simulink model "Model"  (R2018b)
settings: Solver=ode1  StartTime=0.0  StopTime=inf  FixedStep=0.5  RelTol=1e-3
PostLoadFcn:
  | if any(exist('dsrtsu_mdlpostloadfcn', 'file') ~= 0), dsrtsu_mdlpostloadfcn('Execute', bdroot); end
InitFcn:
  | , if any(exist('dsmpb_private', 'file') ~= 0), dsmpb_private('dsmpb_mdlclblib', 'Init', bdroot); end,
  | load('LUT_PSM.mat')
  | load('Torque_ts.mat')
  | 
  | p = 1;
  | L_q = 1.575e-3;
  | L_d = L_q;
  | Psi_M = 0.0353*2*pi;
  | R_s = 639e-3;
  | Ts = 1/25e3;
  | J_ges = 9.56e-5;
  | d_viskos = 0.01;
  | mpsTestMaxVelocityDmd = 166.7;
  | mpsTestVelocityDmd = 0;
  | EDC_CURRENT_CONTROL_EXECUTION_PERIOD = 4e-5;
  | 
undefined symbols (not defined in the file): d, motor_KF, Psidq, Psiqd, q
libraries: dsmpblib x12, simulink x1, simulink_extras x1
(part 2 of 2)

== matlab function Model/DIME Regler/Controller/Decoupling ==
  data: iq input; yd output; p input; w input; Lq input; id input; Ld input; yq output; phi input
function [yd,yq] = fcn(iq,p,w,Lq,id,Ld,phi)

yd= -iq*w*p*Lq;

yq= id*w*p*Ld +phi*p*w;

== matlab function Model/DIME Regler/Controller/MATLAB Function ==
  data: T input; iq output
function iq = fcn(T)
p=1;
Psi_M = 0.0353*2*pi;
iq = T/(3/2* p *Psi_M);

== matlab function Model/DIME Regler/Controller/Identifier_AnyTask/NN Identifier ==
  settings: updateMethod=DISCRETE
  data: h input; id input; iq input; ud input; uq input; omega input; R output; d_id input; d_iq input; Gamma_Theta_R input; Gamma_W_R input; psi_m0 output; J output; Gamma_Theta_psi input; Gamma_W_psi input; takeover input; psim0_est input
function [R, psi_m0, J] = Approximate(h,id,iq,ud,uq,omega, d_id, d_iq, ...
    Gamma_Theta_R, Gamma_W_R,  Gamma_Theta_psi, Gamma_W_psi, takeover, psim0_est )

    % % HRB nominal parameters 
    % Psi_M = 0.0353*2*pi;
    % R_s = 639e-3;


 
if(1)
    Gamma_Theta_ldq10=0;
    Gamma_W_ldq10 = 0;
end
if(1)
    Gamma_Theta_lqd10=0;
    Gamma_W_lqd10 = 0;
end
 




persistent W_R_T ...
           W_l_qd10_T ...
           W_l_dq10_T ...
           W_psi_m0_T ...
           Theta_R_T ...
           Theta_l_qd10_T ...
           Theta_l_dq10_T ...
           Theta_psi_m0_T ...


if isempty(W_R_T) || isempty(W_l_qd10_T) || isempty(W_l_dq10_T) ||  isempty(W_psi_m0_T) || isempty(Theta_R_T) || isempty(Theta_l_qd10_T)  || isempty(Theta_l_dq10_T) ||  isempty(Theta_psi_m0_T)      
 
 
W_R_T = [2.04822644461840e-05,2.04816119048058e-05;2.04823577258696e-05,2.04822462184732e-05;2.04815774888327e-05,2.04817617170584e-05;2.04823629611794e-05,2.04819781184588e-05;2.04820849325778e-05,2.04816182220611e-05;2.04815497917300e-05,2.04820542332664e-05;2.04817290895107e-05,2.04817135625764e-05;2.04819978477042e-05,2.04821050452835e-05;2.04824082972273e-05,2.04821400048950e-05;2.04824137487725e-05,2.04821970118301e-05];
 
Theta_R_T = [0.0179437411497698	0.00897193402779521	0.00897193446402229	0.00897193417960009	0.00897193400199923	0.00897193458740008	0.00897193452389927	0.00897193419739507	0.00897193427267327	0.00897193423924112	0.00897193386022727];
 
W_psi_m0_T = [3.36596323929511e-07,3.35943782551311e-07;3.36687643195459e-07,3.36576135799067e-07;3.35908676332707e-07,3.36092904558458e-07;3.36694960020311e-07,3.36310117299679e-07;3.36414284189910e-07,3.35947573673185e-07;3.35879428791493e-07,3.36383870327895e-07;3.36060197795233e-07,3.36044670860906e-07;3.36328623112877e-07,3.36435820692149e-07;3.36739227973001e-07,3.36470935640707e-07;3.36746389889419e-07,3.36529652947043e-07];
 
Theta_psi_m0_T  = [0.00231788201112145	0.00115894119229074	0.00115894162568093	0.00115894134619483	0.00115894116467780	0.00115894175257942	0.00115894168946356	0.00115894136358532	0.00115894143628631	0.00115894140111420	0.00115894102185007];
 
Theta_l_dq10_T = [3.06272108646170e-05	1.53136618898215e-05	1.53140948664430e-05	1.53138161019030e-05	1.53136340111074e-05	1.53142222806330e-05	1.53141592211266e-05	1.53138334334557e-05	1.53139057572415e-05	1.53138703302795e-05	1.53134910283740e-05];
 
Theta_l_qd10_T = [3.61010730022179e-05	2.24659001336882e-05	2.24663328343095e-05	2.24660542446031e-05	2.24658722745621e-05	2.24664601632891e-05	2.24663971440134e-05	2.24660715653744e-05	2.24661438450041e-05	2.24661084424157e-05	2.24657293848019e-05];
 
W_l_dq10_T = [8.14669546231156e-10,1.62128168031204e-10;9.05741112018515e-10,7.94233715626875e-10;1.26933856909712e-10,3.11162082660982e-10;9.13321502492780e-10,5.28478781859986e-10;6.32309396785878e-10,1.65598880060266e-10;9.74900727413724e-11,6.01931609143709e-10;2.78445392179253e-10,2.62918457852358e-10;5.46829246235578e-10,6.54026825507379e-10;9.57454291187415e-10,6.89161958893324e-10;9.64833086769558e-10,7.48096144394093e-10];
 
W_l_qd10_T = [-0.000643412476326285,-0.000643413128867663;-0.000643412385485832,-0.000643412496993229;-0.000643413163888063,-0.000643412979659837;-0.000643412377824077,-0.000643412762666797;-0.000643412658626792,-0.000643413125337309;-0.000643413193414641,-0.000643412688973105;-0.000643413012409694,-0.000643413027936628;-0.000643412744237816,-0.000643412637040237;-0.000643412333756349,-0.000643412602048681;-0.000643412326400265,-0.000643412543137207];


end

 
x=1;    
 

x_bar = [1,x]';


 
L_q = 1.575e-3;
L_d = L_q;



R      = Theta_R_T      * Phi_1_T( W_R_T * x_bar )  ;

l_qd10 = L_q ;

l_dq10 = L_d ;

psi_m0 = Theta_psi_m0_T * Phi_1_T( W_psi_m0_T * x_bar ) ;

if(takeover)
psi_m0=psim0_est;
end

l_dq20 = 0; 
l_dq30 = 0; 
l_qd30 = 0; 
c_dq01 = 0;  
c_dq11 = 0;  

 
 
ud_hat = R*id - omega * ( l_qd10*iq + l_qd30*iq^3 + c_dq01*id*iq + 0.5*c_dq11*id^2*iq ) + (l_dq10 + 2*l_dq20*id + 3*l_dq30*id^2 + 0.5*c_dq11*iq^2) *  d_id;

uq_hat = R*iq + omega * ( psi_m0 + 0.5*c_dq01*iq^2 + l_dq10*id + l_dq20*id^2 + l_dq30*id^3 + 0.5*c_dq11*id*iq^2 ) + ( l_qd10 + 3*l_qd30*iq^2 + c_dq01*id + 0.5*c_dq11*id^2 ) * d_iq;

J = 0.5 * (ud_hat - ud)^2 + 0.5 * (uq_hat - uq)^2 ;

DJd = ud_hat - ud;
DJq = uq_hat - uq;

 


J_Theta_R_T      = Phi_1_T( W_R_T      * x_bar ) * (DJd * id                                   + DJq * iq);
J_Theta_l_qd10_T = Phi_1_T( W_l_qd10_T * x_bar ) * (DJd * (-omega*iq)                          + DJq * d_iq);
J_Theta_l_dq10_T = Phi_1_T( W_l_dq10_T * x_bar ) * (DJd * ( d_id )                             + DJq * ( id )* omega ) ;
J_Theta_psi_m0_T = Phi_1_T( W_psi_m0_T * x_bar ) * (                                             DJq * ( omega ));

  
J_W_R_T      = x_bar *( Theta_R_T(2:end)      * diag( dsigma( W_R_T      * x_bar ) ) * ( DJd * ( id )                                 + DJq * ( iq ) ) ); % 8x1 * 1x3 = 8x3
J_W_l_qd10_T = x_bar *( Theta_l_qd10_T(2:end) * diag( dsigma( W_l_qd10_T * x_bar ) ) * ( DJd * ( -omega*iq )                          + DJq * ( d_iq ) ) ); 
J_W_l_dq10_T = x_bar *( Theta_l_dq10_T(2:end) * diag( dsigma( W_l_dq10_T * x_bar ) ) * ( DJd * ( d_id )                               + DJq * ( omega*id ) ) ); 
J_W_psi_m0_T = x_bar *( Theta_psi_m0_T(2:end) * diag( dsigma( W_psi_m0_T * x_bar ) ) * (                                                DJq * ( omega ) ) ); 


Theta_R_T      = Theta_R_T      - 5e2*Gamma_Theta_R * J_Theta_R_T'      * h; 
Theta_l_qd10_T = Theta_l_qd10_T -  .2*Gamma_Theta_lqd10 * J_Theta_l_qd10_T'    * h; 
Theta_l_dq10_T = Theta_l_dq10_T -  .00005*Gamma_Theta_ldq10 * J_Theta_l_dq10_T' * h; 
Theta_psi_m0_T = Theta_psi_m0_T - 1*Gamma_Theta_psi * J_Theta_psi_m0_T'   * h;  

 
W_R_T      = W_R_T      - 5e2*Gamma_W_lqd10 * J_W_R_T'      * h; 
W_l_qd10_T = W_l_qd10_T - .2*Gamma_W_R * J_W_l_qd10_T' * h; 
W_l_dq10_T = W_l_dq10_T - .00005*Gamma_W_ldq10 * J_W_l_dq10_T' * h; 
W_psi_m0_T = W_psi_m0_T - 1*Gamma_W_psi * J_W_psi_m0_T' * h; 

  
 


 

function ds = dsigma(x)
a = 1;
ds = a*exp(-a*x)./( 1 + exp(-a*x) ).^2;
end

function Sigma = Phi_1_T(x)
a = 1;
s = 1./( 1 + exp(-a*x) );
Sigma = [1;s];
end

 

 


end

== matlab function Model/DIME Regler/Controller/MATLAB Function1 ==
  data: Udc input; Udc_filt output; Udc_set input
function Udc_filt = fcn(Udc, Udc_set)

if abs(Udc - Udc_set) > 20; 
    Udc_filt = Udc_set; 
else Udc_filt = Udc;
end

== matlab function Model/DIME Regler/Controller/MATLAB Function2 ==
  data: u input; y output; t input
function y = fcn(u,t)

persistent yk uk
if isempty(yk) || isempty(uk)
    uk = 0;
    yk = 0;
end

fc = 1e2;
% t = 5e-7;
T = 1/(2*pi*fc);

a0 = (t/T-1);
b0 = t/T;
% yk + a0 yk-1 = b0 uk-1
yk = -a0 * yk + b0 * uk;

uk = u;
y = yk;

== matlab function Model/DIME Regler/dSpace Measurement/Inc Position Input/Moving Average ==
  data: y input; ymean output
function ymean = fcn( y )
persistent buf n buffull ;
ws = 500 ; % moving average window

% if isempty(buf)
% winSum = zeros(numel(y), 1) ;
% buf = zeros(numel(y), ws) ;
% n = 1 ;
% end
%
% winSum = winSum - buf(:, n) ; % delete oldest value
% winSum = winSum + y ; % add new value
% ymean = winSum ./ min(n, ws) ; % if n ws
% n = 1;
% end

if isempty(n)
n = 1 ;
buf = zeros(numel(y), ws) ;
buffull = 0 ;
end

buf(:, n) = y ;

ymean = y ;
if buffull % averaging only starts after buffer full
ymean = mean(buf, 2) ;
end

n = n + 1;
if n > ws
n = 1 ;
buffull = 1 ;
end

end

== matlab function Model/DIME Regler/Controller/ClarkePark ==
  data: ia input; id output; ib input; ic input; theta input; iq output; ids output; iqs output
function [ id,iq, ids, iqs] = fcn(ia,ib,ic,theta)

ids = (2/3)*( ia - ib/2 -ic/2 );
iqs = (2/3)*(sqrt(3)/2 * ib -  sqrt(3)/2*ic );

 
id = cos(theta)*ids + sin(theta)*iqs;
iq = -sin(theta)*ids + cos(theta)*iqs;
